simulink model "MB_R2018a"  (R2018a)
settings: Solver=VariableStepAuto  StartTime=0.0  StopTime=50  RelTol=1e-3
libraries: simulink x1
settings Model: Creator=win10  LastModifiedBy=tina

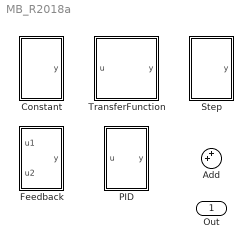
== system MB_R2018a ==
  Add : Sum  Inputs=++|
  Constant : Subsystem  mask{k=1}
  Feedback : Subsystem
  PID : Subsystem  mask{k=1, Ti=1, Td=1}
  Step : Subsystem  mask{startTime=0}
  TransferFunction : Subsystem  mask{b=[1 1], a=[1 1]}
  Out : Outport  VectorParamsAs1DForOutWhenUnconnected=off

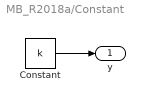
== system MB_R2018a/Constant ==
  Constant : Constant  Value=k
  y : Outport  VectorParamsAs1DForOutWhenUnconnected=off
  wires:
  Constant/1 -> y/1

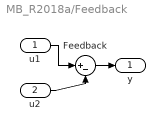
== system MB_R2018a/Feedback ==
  u1 : Inport
  u2 : Inport  Port=2
  Feedback : Sum  Inputs=|+-
  y : Outport  VectorParamsAs1DForOutWhenUnconnected=off
  wires:
  u1/1 -> Feedback/1
  u2/1 -> Feedback/2
  Feedback/1 -> y/1

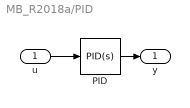
== system MB_R2018a/PID ==
  u : Inport
  PID : simulink/Continuous/PID Controller  Controller=PID  Form=Parallel  TimeDomain=Continuous-time  SampleTime=-1  IntegratorMethod=Forward Euler  FilterMethod=Forward Euler  ControllerParametersSource=internal  P=k  I=Ti  D=Td  UseFilter=on  N=1  TunerSelectOption=Transfer Function Based (PID Tuner App)  InitialConditionSource=internal  InitialConditionForIntegrator=0  InitialConditionForFilter=0  DifferentiatorICPrevScaledInput=0  ExternalReset=none  TrackingMode=off  Kt=1  LimitOutput=off  UpperSaturationLimit=inf  LowerSaturationLimit=-inf  LinearizeAsGain=on  AntiWindupMode=none  Kb=1  POutMin=[]  POutMax=[]  IOutMin=[]  IOutMax=[]  DOutMin=[]  DOutMax=[]  NOutMin=[]  NOutMax=[]  SumOutMin=[]  SumOutMax=[]  SaturationOutMin=[]  SaturationOutMax=[]  PParamMin=[]  PParamMax=[]  IParamMin=[]  IParamMax=[]  DParamMin=[]  DParamMax=[]  NParamMin=[]  NParamMax=[]  KbParamMin=[]  KbParamMax=[]  KtParamMin=[]  KtParamMax=[]  KbOutMin=[]  KbOutMax=[]  KtOutMin=[]  KtOutMax=[]  IntegratorOutMin=[]  IntegratorOutMax=[]  FilterOutMin=[]  FilterOutMax=[]  SumI1OutMin=[]  SumI1OutMax=[]  SumI2OutMin=[]  SumI2OutMax=[]  SumI3OutMin=[]  SumI3OutMax=[]  SumDOutMin=[]  SumDOutMax=[]  DifferentiatorOutMin=[]  DifferentiatorOutMax=[]  FilterDiffOutCoefMin=[]  FilterDiffOutCoefMax=[]  ReciprocalOutMin=[]  ReciprocalOutMax=[]  SumDenOutMin=[]  SumDenOutMax=[]  SumNumOutMin=[]  SumNumOutMax=[]  DivideOutMin=[]  DivideOutMax=[]  IntegratorContinuousStateAttributes=''  IntegratorStateMustResolveToSignalObject=off  IntegratorRTWStateStorageClass=Auto  FilterContinuousStateAttributes=''  FilterStateMustResolveToSignalObject=off  FilterRTWStateStorageClass=Auto
  y : Outport  VectorParamsAs1DForOutWhenUnconnected=off
  wires:
  PID/1 -> y/1
  u/1 -> PID/1

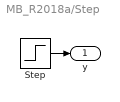
== system MB_R2018a/Step ==
  Step : Step  Time=startTime  SampleTime=0
  y : Outport  VectorParamsAs1DForOutWhenUnconnected=off
  wires:
  Step/1 -> y/1

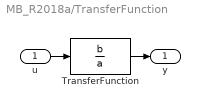
== system MB_R2018a/TransferFunction ==
  u : Inport
  TransferFunction : TransferFcn  Numerator=b  Denominator=a
  y : Outport  VectorParamsAs1DForOutWhenUnconnected=off
  wires:
  TransferFunction/1 -> y/1
  u/1 -> TransferFunction/1
